simulink model "RLCprimaEserci"  (R2018b)
settings: Solver=VariableStepAuto  StartTime=0.0  StopTime=0.02  MaxStep=1e-7  RelTol=1e-3
values from neighbouring files (symbols this model uses):
  C = [ 1 -1]    [esercizio2.m]    (also in rlc.m = 1e-06; stabilita.m = [ 1 0 3])
  L = 1e-3    (= 0.001)    [rlc.m]
  R = 0    [SIR.m]    (also in exe_vari_regressioe_autoval.m = chol(A_1); prova esame.m = chol(B); rlc.m; soluzioni_3.m = chol(A))
settings Model: Creator=Antonella  LastModifiedBy=Antonella

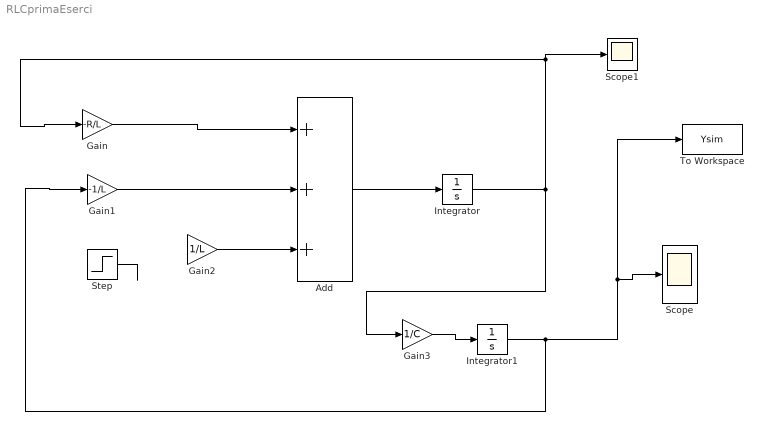
== system RLCprimaEserci ==
  Add : Sum  Inputs=+++
  Gain : Gain  Gain=-R/L
  Gain1 : Gain  Gain=-1/L
  Gain2 : Gain  Gain=1/L
  Gain3 : Gain  Gain=1/C
  Integrator : Integrator  InitialCondition=20e-3
  Integrator1 : Integrator  InitialCondition=3
  Scope : Scope
  Scope1 : Scope
  Step : Step  Time=0  SampleTime=0
  To Workspace : ToWorkspace  VariableName=Ysim  SaveFormat=Structure With Time  SampleTime=-1
  wires:
  Gain2/1 -> Add/3
  Gain1/1 -> Add/2
  Gain/1 -> Add/1
  Add/1 -> Integrator/1
  Step/1 -> ?
  Integrator/1 -> Scope1/1, Gain/1, Gain3/1
  Gain3/1 -> Integrator1/1
  Integrator1/1 -> To Workspace/1, Scope/1, Gain1/1
